simulink model "memristors_LSTM"  (R2020b)
settings: Solver=VariableStepAuto  StartTime=0.0  StopTime=3  RelTol=1e-3
libraries: simulink x17
(part 1 of 5)
settings Model: Creator=Иван  LastModifiedBy=Иван

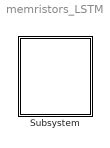
== system memristors_LSTM ==
  Subsystem : Subsystem

== system memristors_LSTM/Subsystem ==
  Add : Sum
  Display : Display
  Memristor crossbar1 : Subsystem
  Memristor crossbar2 : Subsystem
  Memristor crossbar4 : Subsystem
  Product : Product
  Product1 : Product
  Product2 : Product
  SIG : Subsystem
  SIG1 : Subsystem
  SIG2 : Subsystem
  TANH : Subsystem
  TANH1 : Subsystem
  s : Subsystem
  wires:
  Product/1 -> Add/1
  Product1/1 -> Add/2
  TANH1/1(Out1) -> Product2/2
  SIG2/1(Out1) -> Product2/1
  TANH/1(Out1) -> Product1/2
  SIG1/1(Out1) -> Product1/1
  Add/1 -> TANH1/1(In1)
  Memristor crossbar2/1(Out1) -> SIG1/1(In1)
  s/1(Out1) -> TANH/1(In1)
  Memristor crossbar4/1(Out1) -> SIG2/1(In1)
  Product2/1 -> Display/1
  SIG/1(Out1) -> Product/1
  Memristor crossbar1/1(Out1) -> SIG/1(In1)

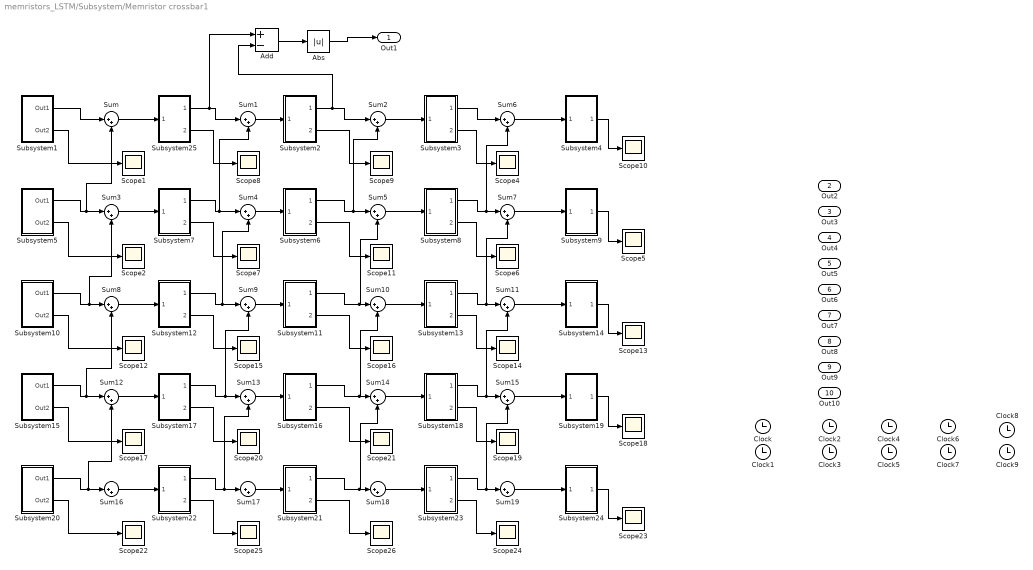
== system memristors_LSTM/Subsystem/Memristor crossbar1 ==
  Abs : Abs
  Add : Sum  Inputs=+-
  Clock{,1..9} (10 alike) : Clock
  Scope{1..2,4..26} (25 alike) : Scope
  Subsystem1 : Subsystem
  Subsystem10 : Subsystem
  Subsystem11 : Subsystem
  Subsystem12 : Subsystem
  Subsystem13 : Subsystem
  Subsystem14 : Subsystem
  Subsystem15 : Subsystem
  Subsystem16 : Subsystem
  Subsystem17 : Subsystem
  Subsystem18 : Subsystem
  Subsystem19 : Subsystem
  Subsystem2 : Subsystem
  Subsystem20 : Subsystem
  Subsystem21 : Subsystem
  Subsystem22 : Subsystem
  Subsystem23 : Subsystem
  Subsystem24 : Subsystem
  Subsystem25 : Subsystem
  Subsystem3 : Subsystem
  Subsystem4 : Subsystem
  Subsystem5 : Subsystem
  Subsystem6 : Subsystem
  Subsystem7 : Subsystem
  Subsystem8 : Subsystem
  Subsystem9 : Subsystem
  Sum{,1..19} (20 alike) : Sum  Inputs=|++
  Out1 : Outport
  Out2 : Outport  Port=2
  Out3 : Outport  Port=3
  Out4 : Outport  Port=4
  Out5 : Outport  Port=5
  Out6 : Outport  Port=6
  Out7 : Outport  Port=7
  Out8 : Outport  Port=8
  Out9 : Outport  Port=9
  Out10 : Outport  Port=10
  wires:
  Subsystem8/1(Out1) -> Sum6/2, Sum7/1
  Subsystem23/2(Out2) -> Scope24/1
  Subsystem6/1(Out1) -> Sum2/2, Sum5/1
  Subsystem20/1(Out1) -> Sum12/2, Sum16/1
  Subsystem1/1(Out1) -> Sum/1
  Subsystem2/1(Out1) -> Add/2, Sum2/1
  Subsystem17/2(Out2) -> Scope20/1
  Subsystem7/1(Out1) -> Sum1/2, Sum4/1
  Sum1/1 -> Subsystem2/1(In1)
  Subsystem18/1(Out1) -> Sum11/2, Sum15/1
  Subsystem6/2(Out2) -> Scope11/1
  Sum4/1 -> Subsystem6/1(In1)
  Subsystem5/2(Out2) -> Scope2/1
  Subsystem18/2(Out2) -> Scope19/1
  Subsystem11/1(Out1) -> Sum5/2, Sum10/1
  Sum18/1 -> Subsystem23/1(In1)
  Subsystem17/1(Out1) -> Sum9/2, Sum13/1
  Subsystem25/2(Out2) -> Scope8/1
  Subsystem13/2(Out2) -> Scope14/1
  Sum11/1 -> Subsystem14/1(In1)
  Subsystem21/2(Out2) -> Scope26/1
  Sum17/1 -> Subsystem21/1(In1)
  Sum/1 -> Subsystem25/1(In1)
  Subsystem2/2(Out2) -> Scope9/1
  Subsystem1/2(Out2) -> Scope1/1
  Subsystem20/2(Out2) -> Scope22/1
  Subsystem25/1(Out1) -> Add/1, Sum1/1
  Sum15/1 -> Subsystem19/1(In1)
  Sum8/1 -> Subsystem12/1(In1)
  Subsystem4/1(Out2) -> Scope10/1
  Subsystem5/1(Out1) -> Sum/2, Sum3/1
  Subsystem22/1(Out1) -> Sum13/2, Sum17/1
  Subsystem11/2(Out2) -> Scope16/1
  Sum5/1 -> Subsystem8/1(In1)
  Subsystem10/1(Out1) -> Sum3/2, Sum8/1
  Subsystem8/2(Out2) -> Scope6/1
  Subsystem7/2(Out2) -> Scope7/1
  Sum13/1 -> Subsystem16/1(In1)
  Subsystem10/2(Out2) -> Scope12/1
  Subsystem15/1(Out1) -> Sum8/2, Sum12/1
  Subsystem12/1(Out1) -> Sum4/2, Sum9/1
  Sum9/1 -> Subsystem11/1(In1)
  Sum6/1 -> Subsystem4/1(In1)
  Subsystem16/2(Out2) -> Scope21/1
  Subsystem13/1(Out1) -> Sum7/2, Sum11/1
  Sum19/1 -> Subsystem24/1(In1)
  Subsystem3/2(Out2) -> Scope4/1
  Sum7/1 -> Subsystem9/1(In1)
  Subsystem14/1(Out2) -> Scope13/1
  Subsystem16/1(Out1) -> Sum10/2, Sum14/1
  Subsystem3/1(Out1) -> Sum6/1
  Subsystem22/2(Out2) -> Scope25/1
  Sum12/1 -> Subsystem17/1(In1)
  Subsystem24/1(Out2) -> Scope23/1
  Subsystem9/1(Out2) -> Scope5/1
  Subsystem15/2(Out2) -> Scope17/1
  Sum10/1 -> Subsystem13/1(In1)
  Subsystem23/1(Out1) -> Sum15/2, Sum19/1
  Sum2/1 -> Subsystem3/1(In1)
  Subsystem12/2(Out2) -> Scope15/1
  Subsystem19/1(Out2) -> Scope18/1
  Sum14/1 -> Subsystem18/1(In1)
  Sum3/1 -> Subsystem7/1(In1)
  Subsystem21/1(Out1) -> Sum14/2, Sum18/1
  Sum16/1 -> Subsystem22/1(In1)
  Add/1 -> Abs/1
  Abs/1 -> Out1/1

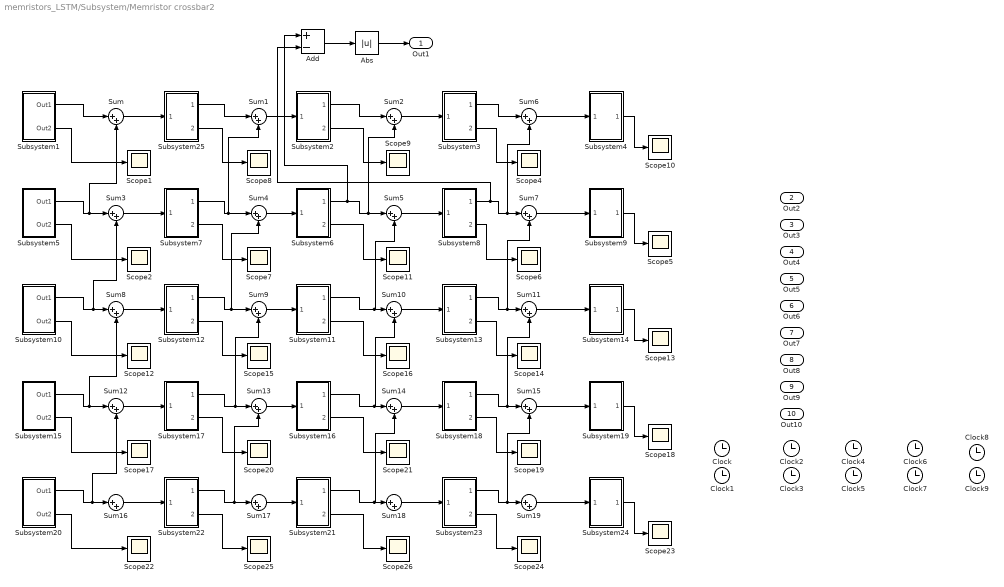
== system memristors_LSTM/Subsystem/Memristor crossbar2 ==
  Abs : Abs
  Add : Sum  Inputs=+-
  Clock{,1..9} (10 alike) : Clock
  Scope{1..2,4..26} (25 alike) : Scope
  Subsystem1 : Subsystem
  Subsystem10 : Subsystem
  Subsystem11 : Subsystem
  Subsystem12 : Subsystem
  Subsystem13 : Subsystem
  Subsystem14 : Subsystem
  Subsystem15 : Subsystem
  Subsystem16 : Subsystem
  Subsystem17 : Subsystem
  Subsystem18 : Subsystem
  Subsystem19 : Subsystem
  Subsystem2 : Subsystem
  Subsystem20 : Subsystem
  Subsystem21 : Subsystem
  Subsystem22 : Subsystem
  Subsystem23 : Subsystem
  Subsystem24 : Subsystem
  Subsystem25 : Subsystem
  Subsystem3 : Subsystem
  Subsystem4 : Subsystem
  Subsystem5 : Subsystem
  Subsystem6 : Subsystem
  Subsystem7 : Subsystem
  Subsystem8 : Subsystem
  Subsystem9 : Subsystem
  Sum{,1..19} (20 alike) : Sum  Inputs=|++
  Out1 : Outport
  Out2 : Outport  Port=2
  Out3 : Outport  Port=3
  Out4 : Outport  Port=4
  Out5 : Outport  Port=5
  Out6 : Outport  Port=6
  Out7 : Outport  Port=7
  Out8 : Outport  Port=8
  Out9 : Outport  Port=9
  Out10 : Outport  Port=10
  wires:
  Subsystem8/1(Out1) -> Add/2, Sum6/2, Sum7/1
  Subsystem23/2(Out2) -> Scope24/1
  Subsystem6/1(Out1) -> Add/1, Sum2/2, Sum5/1
  Subsystem20/1(Out1) -> Sum12/2, Sum16/1
  Subsystem1/1(Out1) -> Sum/1
  Subsystem2/1(Out1) -> Sum2/1
  Subsystem17/2(Out2) -> Scope20/1
  Subsystem7/1(Out1) -> Sum1/2, Sum4/1
  Sum1/1 -> Subsystem2/1(In1)
  Subsystem18/1(Out1) -> Sum11/2, Sum15/1
  Subsystem6/2(Out2) -> Scope11/1
  Sum4/1 -> Subsystem6/1(In1)
  Subsystem5/2(Out2) -> Scope2/1
  Subsystem18/2(Out2) -> Scope19/1
  Subsystem11/1(Out1) -> Sum5/2, Sum10/1
  Sum18/1 -> Subsystem23/1(In1)
  Subsystem17/1(Out1) -> Sum9/2, Sum13/1
  Subsystem25/2(Out2) -> Scope8/1
  Subsystem13/2(Out2) -> Scope14/1
  Sum11/1 -> Subsystem14/1(In1)
  Subsystem21/2(Out2) -> Scope26/1
  Sum17/1 -> Subsystem21/1(In1)
  Sum/1 -> Subsystem25/1(In1)
  Subsystem2/2(Out2) -> Scope9/1
  Subsystem1/2(Out2) -> Scope1/1
  Subsystem20/2(Out2) -> Scope22/1
  Subsystem25/1(Out1) -> Sum1/1
  Sum15/1 -> Subsystem19/1(In1)
  Sum8/1 -> Subsystem12/1(In1)
  Subsystem4/1(Out2) -> Scope10/1
  Subsystem5/1(Out1) -> Sum/2, Sum3/1
  Subsystem22/1(Out1) -> Sum13/2, Sum17/1
  Subsystem11/2(Out2) -> Scope16/1
  Sum5/1 -> Subsystem8/1(In1)
  Subsystem10/1(Out1) -> Sum3/2, Sum8/1
  Subsystem8/2(Out2) -> Scope6/1
  Subsystem7/2(Out2) -> Scope7/1
  Sum13/1 -> Subsystem16/1(In1)
  Subsystem10/2(Out2) -> Scope12/1
  Subsystem15/1(Out1) -> Sum8/2, Sum12/1
  Subsystem12/1(Out1) -> Sum4/2, Sum9/1
  Sum9/1 -> Subsystem11/1(In1)
  Sum6/1 -> Subsystem4/1(In1)
  Subsystem16/2(Out2) -> Scope21/1
  Subsystem13/1(Out1) -> Sum7/2, Sum11/1
  Sum19/1 -> Subsystem24/1(In1)
  Subsystem3/2(Out2) -> Scope4/1
  Sum7/1 -> Subsystem9/1(In1)
  Subsystem14/1(Out2) -> Scope13/1
  Subsystem16/1(Out1) -> Sum10/2, Sum14/1
  Subsystem3/1(Out1) -> Sum6/1
  Subsystem22/2(Out2) -> Scope25/1
  Sum12/1 -> Subsystem17/1(In1)
  Subsystem24/1(Out2) -> Scope23/1
  Subsystem9/1(Out2) -> Scope5/1
  Subsystem15/2(Out2) -> Scope17/1
  Sum10/1 -> Subsystem13/1(In1)
  Subsystem23/1(Out1) -> Sum15/2, Sum19/1
  Sum2/1 -> Subsystem3/1(In1)
  Subsystem12/2(Out2) -> Scope15/1
  Subsystem19/1(Out2) -> Scope18/1
  Sum14/1 -> Subsystem18/1(In1)
  Sum3/1 -> Subsystem7/1(In1)
  Subsystem21/1(Out1) -> Sum14/2, Sum18/1
  Sum16/1 -> Subsystem22/1(In1)
  Add/1 -> Abs/1
  Abs/1 -> Out1/1

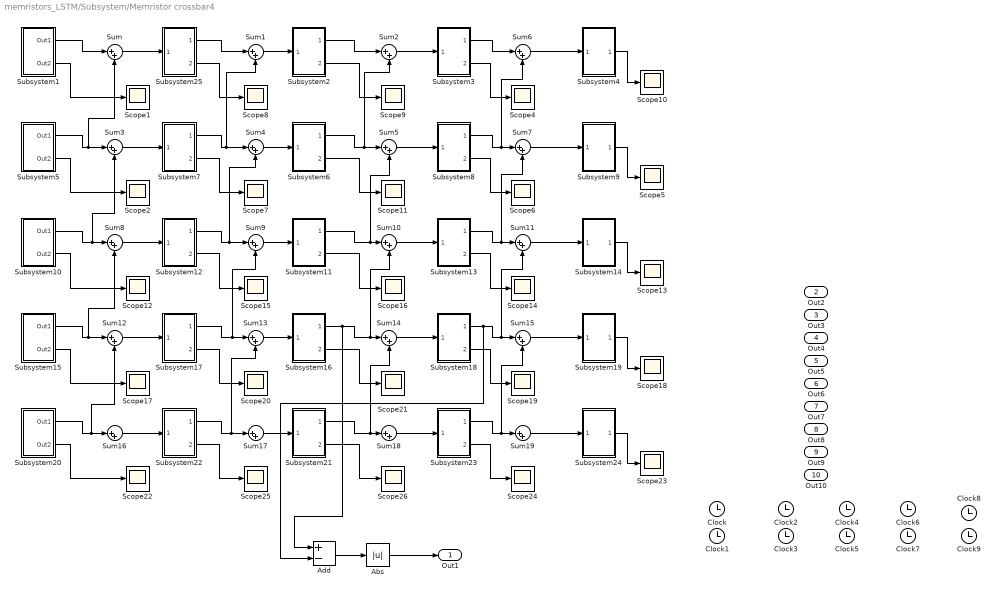
== system memristors_LSTM/Subsystem/Memristor crossbar4 ==
  Abs : Abs
  Add : Sum  Inputs=+-
  Clock{,1..9} (10 alike) : Clock
  Scope{1..2,4..26} (25 alike) : Scope
  Subsystem1 : Subsystem
  Subsystem10 : Subsystem
  Subsystem11 : Subsystem
  Subsystem12 : Subsystem
  Subsystem13 : Subsystem
  Subsystem14 : Subsystem
  Subsystem15 : Subsystem
  Subsystem16 : Subsystem
  Subsystem17 : Subsystem
  Subsystem18 : Subsystem
  Subsystem19 : Subsystem
  Subsystem2 : Subsystem
  Subsystem20 : Subsystem
  Subsystem21 : Subsystem
  Subsystem22 : Subsystem
  Subsystem23 : Subsystem
  Subsystem24 : Subsystem
  Subsystem25 : Subsystem
  Subsystem3 : Subsystem
  Subsystem4 : Subsystem
  Subsystem5 : Subsystem
  Subsystem6 : Subsystem
  Subsystem7 : Subsystem
  Subsystem8 : Subsystem
  Subsystem9 : Subsystem
  Sum{,1..19} (20 alike) : Sum  Inputs=|++
  Out1 : Outport
  Out2 : Outport  Port=2
  Out3 : Outport  Port=3
  Out4 : Outport  Port=4
  Out5 : Outport  Port=5
  Out6 : Outport  Port=6
  Out7 : Outport  Port=7
  Out8 : Outport  Port=8
  Out9 : Outport  Port=9
  Out10 : Outport  Port=10
  wires:
  Subsystem8/1(Out1) -> Sum6/2, Sum7/1
  Subsystem23/2(Out2) -> Scope24/1
  Subsystem6/1(Out1) -> Sum2/2, Sum5/1
  Subsystem20/1(Out1) -> Sum12/2, Sum16/1
  Subsystem1/1(Out1) -> Sum/1
  Subsystem2/1(Out1) -> Sum2/1
  Subsystem17/2(Out2) -> Scope20/1
  Subsystem7/1(Out1) -> Sum1/2, Sum4/1
  Sum1/1 -> Subsystem2/1(In1)
  Subsystem18/1(Out1) -> Add/2, Sum11/2, Sum15/1
  Subsystem6/2(Out2) -> Scope11/1
  Sum4/1 -> Subsystem6/1(In1)
  Subsystem5/2(Out2) -> Scope2/1
  Subsystem18/2(Out2) -> Scope19/1
  Subsystem11/1(Out1) -> Sum5/2, Sum10/1
  Sum18/1 -> Subsystem23/1(In1)
  Subsystem17/1(Out1) -> Sum9/2, Sum13/1
  Subsystem25/2(Out2) -> Scope8/1
  Subsystem13/2(Out2) -> Scope14/1
  Sum11/1 -> Subsystem14/1(In1)
  Subsystem21/2(Out2) -> Scope26/1
  Sum17/1 -> Subsystem21/1(In1)
  Sum/1 -> Subsystem25/1(In1)
  Subsystem2/2(Out2) -> Scope9/1
  Subsystem1/2(Out2) -> Scope1/1
  Subsystem20/2(Out2) -> Scope22/1
  Subsystem25/1(Out1) -> Sum1/1
  Sum15/1 -> Subsystem19/1(In1)
  Sum8/1 -> Subsystem12/1(In1)
  Subsystem4/1(Out2) -> Scope10/1
  Subsystem5/1(Out1) -> Sum/2, Sum3/1
  Subsystem22/1(Out1) -> Sum13/2, Sum17/1
  Subsystem11/2(Out2) -> Scope16/1
  Sum5/1 -> Subsystem8/1(In1)
  Subsystem10/1(Out1) -> Sum3/2, Sum8/1
  Subsystem8/2(Out2) -> Scope6/1
  Subsystem7/2(Out2) -> Scope7/1
  Sum13/1 -> Subsystem16/1(In1)
  Subsystem10/2(Out2) -> Scope12/1
  Subsystem15/1(Out1) -> Sum8/2, Sum12/1
  Subsystem12/1(Out1) -> Sum4/2, Sum9/1
  Sum9/1 -> Subsystem11/1(In1)
  Sum6/1 -> Subsystem4/1(In1)
  Subsystem16/2(Out2) -> Scope21/1
  Subsystem13/1(Out1) -> Sum7/2, Sum11/1
  Sum19/1 -> Subsystem24/1(In1)
  Subsystem3/2(Out2) -> Scope4/1
  Sum7/1 -> Subsystem9/1(In1)
  Subsystem14/1(Out2) -> Scope13/1
  Subsystem16/1(Out1) -> Add/1, Sum10/2, Sum14/1
  Subsystem3/1(Out1) -> Sum6/1
  Subsystem22/2(Out2) -> Scope25/1
  Sum12/1 -> Subsystem17/1(In1)
  Subsystem24/1(Out2) -> Scope23/1
  Subsystem9/1(Out2) -> Scope5/1
  Subsystem15/2(Out2) -> Scope17/1
  Sum10/1 -> Subsystem13/1(In1)
  Subsystem23/1(Out1) -> Sum15/2, Sum19/1
  Sum2/1 -> Subsystem3/1(In1)
  Subsystem12/2(Out2) -> Scope15/1
  Subsystem19/1(Out2) -> Scope18/1
  Sum14/1 -> Subsystem18/1(In1)
  Sum3/1 -> Subsystem7/1(In1)
  Subsystem21/1(Out1) -> Sum14/2, Sum18/1
  Sum16/1 -> Subsystem22/1(In1)
  Add/1 -> Abs/1
  Abs/1 -> Out1/1

== system memristors_LSTM/Subsystem/SIG ==
  In1 : Inport
  Add4 : Sum
  Constant1 : Constant
  Constant2 : Constant
  Divide2 : Product  Inputs=*/
  Integrator2 : Integrator  InitialCondition=-10
  Math Function2 : Math  Operator=reciprocal  SaturateOnIntegerOverflow=on
  Math Function3 : Math  SaturateOnIntegerOverflow=on
  Product : Product
  Ramp : simulink/Sources/Ramp  slope=1  start=-4  InitialOutput=0
  Scope1 : Scope
  Out1 : Outport
  wires:
  Constant2/1 -> Add4/1
  Divide2/1 -> Product/1
  Math Function2/1 -> Add4/2
  Math Function3/1 -> Math Function2/1
  Add4/1 -> Divide2/2
  Constant1/1 -> Divide2/1
  Integrator2/1 -> Math Function3/1
  Ramp/1 -> Scope1/1, Integrator2/1
  In1/1 -> Product/2
  Product/1 -> Out1/1

== system memristors_LSTM/Subsystem/SIG1 ==
  In1 : Inport
  Add4 : Sum
  Constant1 : Constant
  Constant2 : Constant
  Divide2 : Product  Inputs=*/
  Integrator2 : Integrator  InitialCondition=-10
  Math Function2 : Math  Operator=reciprocal  SaturateOnIntegerOverflow=on
  Math Function3 : Math  SaturateOnIntegerOverflow=on
  Product : Product
  Ramp : simulink/Sources/Ramp  slope=1  start=-4  InitialOutput=0
  Out1 : Outport
  wires:
  Constant2/1 -> Add4/1
  Math Function2/1 -> Add4/2
  Math Function3/1 -> Math Function2/1
  Integrator2/1 -> Math Function3/1
  Add4/1 -> Divide2/2
  Constant1/1 -> Divide2/1
  Ramp/1 -> Integrator2/1
  Divide2/1 -> Product/2
  In1/1 -> Product/1  "In"
  Product/1 -> Out1/1

== system memristors_LSTM/Subsystem/SIG2 ==
  In1 : Inport
  Add4 : Sum
  Constant1 : Constant
  Constant2 : Constant
  Divide2 : Product  Inputs=*/
  Integrator2 : Integrator  InitialCondition=-10
  Math Function2 : Math  Operator=reciprocal  SaturateOnIntegerOverflow=on
  Math Function3 : Math  SaturateOnIntegerOverflow=on
  Product : Product
  Ramp : simulink/Sources/Ramp  slope=1  start=-4  InitialOutput=0
  Out1 : Outport
  wires:
  Constant2/1 -> Add4/1
  Math Function2/1 -> Add4/2
  Math Function3/1 -> Math Function2/1
  Integrator2/1 -> Math Function3/1
  Add4/1 -> Divide2/2
  Constant1/1 -> Divide2/1
  Ramp/1 -> Integrator2/1
  Divide2/1 -> Product/2
  Product/1 -> Out1/1
  In1/1 -> Product/1

== system memristors_LSTM/Subsystem/TANH ==
  In1 : Inport
  Atanh1 : Trigonometry  Operator=tanh
  Integrator1 : Integrator  InitialCondition=-4
  Product : Product
  Ramp : simulink/Sources/Ramp  slope=1  start=-4  InitialOutput=0
  Out1 : Outport
  wires:
  Ramp/1 -> Integrator1/1
  Integrator1/1 -> Atanh1/1
  Product/1 -> Out1/1
  Atanh1/1 -> Product/2
  In1/1 -> Product/1

== system memristors_LSTM/Subsystem/TANH1 ==
  In1 : Inport
  Atanh1 : Trigonometry  Operator=tanh
  Integrator1 : Integrator  InitialCondition=-4
  Product1 : Product
  Ramp : simulink/Sources/Ramp  slope=1  start=-4  InitialOutput=0
  Scope : Scope
  Out1 : Outport
  wires:
  Atanh1/1 -> Scope/1, Product1/2
  Integrator1/1 -> Atanh1/1
  Ramp/1 -> Integrator1/1
  Product1/1 -> Out1/1
  In1/1 -> Product1/1

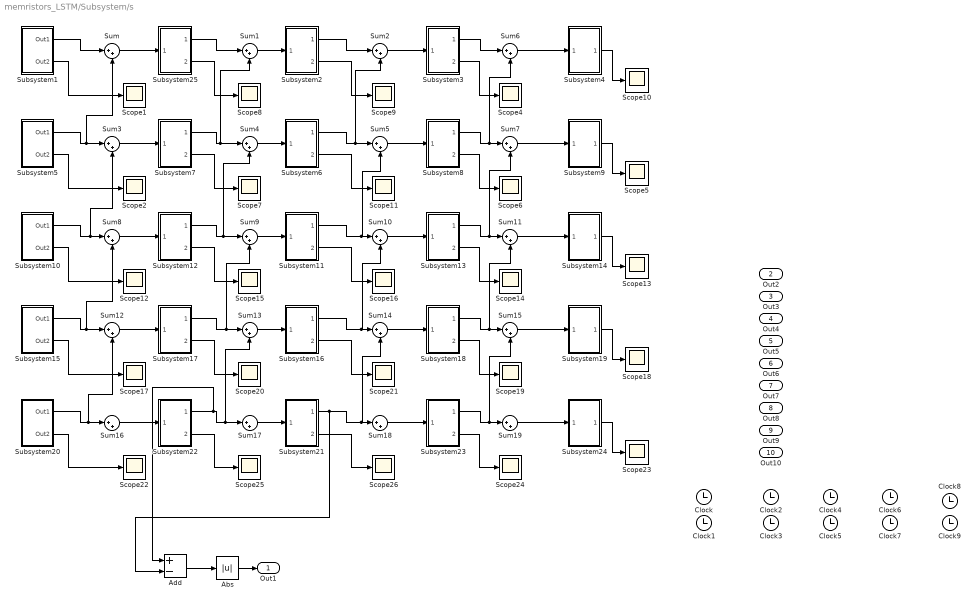
== system memristors_LSTM/Subsystem/s ==
  Abs : Abs
  Add : Sum  Inputs=+-
  Clock{,1..9} (10 alike) : Clock
  Scope{1..2,4..26} (25 alike) : Scope
  Subsystem1 : Subsystem
  Subsystem10 : Subsystem
  Subsystem11 : Subsystem
  Subsystem12 : Subsystem
  Subsystem13 : Subsystem
  Subsystem14 : Subsystem
  Subsystem15 : Subsystem
  Subsystem16 : Subsystem
  Subsystem17 : Subsystem
  Subsystem18 : Subsystem
  Subsystem19 : Subsystem
  Subsystem2 : Subsystem
  Subsystem20 : Subsystem
  Subsystem21 : Subsystem
  Subsystem22 : Subsystem
  Subsystem23 : Subsystem
  Subsystem24 : Subsystem
  Subsystem25 : Subsystem
  Subsystem3 : Subsystem
  Subsystem4 : Subsystem
  Subsystem5 : Subsystem
  Subsystem6 : Subsystem
  Subsystem7 : Subsystem
  Subsystem8 : Subsystem
  Subsystem9 : Subsystem
  Sum{,1..19} (20 alike) : Sum  Inputs=|++
  Out1 : Outport
  Out2 : Outport  Port=2
  Out3 : Outport  Port=3
  Out4 : Outport  Port=4
  Out5 : Outport  Port=5
  Out6 : Outport  Port=6
  Out7 : Outport  Port=7
  Out8 : Outport  Port=8
  Out9 : Outport  Port=9
  Out10 : Outport  Port=10
  wires:
  Subsystem8/1(Out1) -> Sum6/2, Sum7/1
  Subsystem23/2(Out2) -> Scope24/1
  Subsystem6/1(Out1) -> Sum2/2, Sum5/1
  Subsystem20/1(Out1) -> Sum12/2, Sum16/1
  Subsystem1/1(Out1) -> Sum/1
  Subsystem2/1(Out1) -> Sum2/1
  Subsystem17/2(Out2) -> Scope20/1
  Subsystem7/1(Out1) -> Sum1/2, Sum4/1
  Sum1/1 -> Subsystem2/1(In1)
  Subsystem18/1(Out1) -> Sum11/2, Sum15/1
  Subsystem6/2(Out2) -> Scope11/1
  Sum4/1 -> Subsystem6/1(In1)
  Subsystem5/2(Out2) -> Scope2/1
  Subsystem18/2(Out2) -> Scope19/1
  Subsystem11/1(Out1) -> Sum5/2, Sum10/1
  Sum18/1 -> Subsystem23/1(In1)
  Subsystem17/1(Out1) -> Sum9/2, Sum13/1
  Subsystem25/2(Out2) -> Scope8/1
  Subsystem13/2(Out2) -> Scope14/1
  Sum11/1 -> Subsystem14/1(In1)
  Subsystem21/2(Out2) -> Scope26/1
  Sum17/1 -> Subsystem21/1(In1)
  Sum/1 -> Subsystem25/1(In1)
  Subsystem2/2(Out2) -> Scope9/1
  Subsystem1/2(Out2) -> Scope1/1
  Subsystem20/2(Out2) -> Scope22/1
  Subsystem25/1(Out1) -> Sum1/1
  Sum15/1 -> Subsystem19/1(In1)
  Sum8/1 -> Subsystem12/1(In1)
  Subsystem4/1(Out2) -> Scope10/1
  Subsystem5/1(Out1) -> Sum/2, Sum3/1
  Subsystem22/1(Out1) -> Add/1, Sum13/2, Sum17/1
  Subsystem11/2(Out2) -> Scope16/1
  Sum5/1 -> Subsystem8/1(In1)
  Subsystem10/1(Out1) -> Sum3/2, Sum8/1
  Subsystem8/2(Out2) -> Scope6/1
  Subsystem7/2(Out2) -> Scope7/1
  Sum13/1 -> Subsystem16/1(In1)
  Subsystem10/2(Out2) -> Scope12/1
  Subsystem15/1(Out1) -> Sum8/2, Sum12/1
  Subsystem12/1(Out1) -> Sum4/2, Sum9/1
  Sum9/1 -> Subsystem11/1(In1)
  Sum6/1 -> Subsystem4/1(In1)
  Subsystem16/2(Out2) -> Scope21/1
  Subsystem13/1(Out1) -> Sum7/2, Sum11/1
  Sum19/1 -> Subsystem24/1(In1)
  Subsystem3/2(Out2) -> Scope4/1
  Sum7/1 -> Subsystem9/1(In1)
  Subsystem14/1(Out2) -> Scope13/1
  Subsystem16/1(Out1) -> Sum10/2, Sum14/1
  Subsystem3/1(Out1) -> Sum6/1
  Subsystem22/2(Out2) -> Scope25/1
  Sum12/1 -> Subsystem17/1(In1)
  Subsystem24/1(Out2) -> Scope23/1
  Subsystem9/1(Out2) -> Scope5/1
  Subsystem15/2(Out2) -> Scope17/1
  Sum10/1 -> Subsystem13/1(In1)
  Subsystem23/1(Out1) -> Sum15/2, Sum19/1
  Sum2/1 -> Subsystem3/1(In1)
  Subsystem12/2(Out2) -> Scope15/1
  Subsystem19/1(Out2) -> Scope18/1
  Sum14/1 -> Subsystem18/1(In1)
  Sum3/1 -> Subsystem7/1(In1)
  Subsystem21/1(Out1) -> Add/2, Sum14/2, Sum18/1
  Sum16/1 -> Subsystem22/1(In1)
  Add/1 -> Abs/1
  Abs/1 -> Out1/1

== system memristors_LSTM/Subsystem/Memristor crossbar1/Subsystem1 ==
  note: Memristor
  note: k
  note: for I-V
  note: Rmem
  note: f(x)
  note: for x
  note: for processing
  " V" : Sin  Amplitude=0.1  Frequency=0.5  SampleTime=0
  2p : Gain  Gain=2
  2x : Gain  Gain=2
  Add : Sum  Inputs=-+
  Add1 : Sum
  Add2 : Sum  Inputs=-+
  Add3 : Sum  Inputs=+-
  Constant : Constant
  Constant10 : Constant  Value=0
  Constant4 : Constant
  Constant9 : Constant
  D : Constant  Value=10^(-8)
  Divide : Product  Inputs=*/
  Divide1 : Product  Inputs=**/
  Gain2 : Gain
  I-t : Scope
  Integrator : Integrator
  Integrator Initial condition source : Integrator  InitialConditionSource=external
  Math Function : Math  Operator=pow  SaturateOnIntegerOverflow=on
  Math Function1 : Math  Operator=square  SaturateOnIntegerOverflow=on
  Product1 : Product
  Product2 : Product
  Product3 : Product  Inputs=3
  Product4 : Product
  R_off : Constant  Value=20000
  R_on : Constant  Value=100
  R_on1 : Constant  Value=100
  Switch : Switch  Threshold=1
  Switch1 : Switch
  V-t : Scope
  XY Graph : simulink/Sinks/XY Graph  xmin=-0.05  xmax=0.05  ymin=-0.01  ymax=0.01  st=-1
  p : Constant  Value=10
  x-t : Scope
  x0 : Constant  Value=0.7
  𝜇_𝑣 : Constant  Value=10^(-14)
  Out1 : Outport
  Out2 : Outport  Port=2
  wires:
  Constant9/1 -> Switch/1
  Switch/1 -> Switch1/2, Switch1/1
  R_on/1 -> Divide1/1
  Integrator Initial condition source/1 -> Switch/3, Switch/2, x-t/1
  Integrator/1 -> Divide/1, Product4/2
  2p/1 -> Math Function/2
  Divide/1 -> XY Graph/2, I-t/1, Product3/1
  Switch1/1 -> Product2/2, Add/1, 2x/1
  𝜇_𝑣/1 -> Divide1/2
  Gain2/1 -> Integrator/1
  Math Function/1 -> Add3/2
  Add/1 -> Product1/1
  R_on1/1 -> Product2/1
  Constant/1 -> Add/2
  p/1 -> 2p/1
  D/1 -> Math Function1/1
  Divide1/1 -> Product3/3
  2x/1 -> Add2/2
  Product1/1 -> Add1/2
  R_off/1 -> Product1/2
  Add2/1 -> Math Function/1
  Constant4/1 -> Add3/1, Add2/1
  Product4/1 -> Out1/1, XY Graph/1, Out2/1, V-t/1
  Product2/1 -> Add1/1
  x0/1 -> Integrator Initial condition source/2
  Constant10/1 -> Switch1/3
  Product3/1 -> Integrator Initial condition source/1
  Add1/1 -> Divide/2
  Add3/1 -> Product3/2
  Math Function1/1 -> Divide1/3
  " V"/1 -> Gain2/1, Product4/1

== system memristors_LSTM/Subsystem/Memristor crossbar1/Subsystem10 ==
  note: Memristor
  note: k
  note: for I-V
  note: Rmem
  note: f(x)
  note: for x
  note: for processing
  " V" : Sin  Amplitude=0.1  Frequency=0.5  SampleTime=0
  2p : Gain  Gain=2
  2x : Gain  Gain=2
  Add : Sum  Inputs=-+
  Add1 : Sum
  Add2 : Sum  Inputs=-+
  Add3 : Sum  Inputs=+-
  Constant : Constant
  Constant10 : Constant  Value=0
  Constant4 : Constant
  Constant9 : Constant
  D : Constant  Value=10^(-8)
  Divide : Product  Inputs=*/
  Divide1 : Product  Inputs=**/
  Gain2 : Gain  Gain=0.5
  I-t : Scope
  Integrator : Integrator
  Integrator Initial condition source : Integrator  InitialConditionSource=external
  Math Function : Math  Operator=pow  SaturateOnIntegerOverflow=on
  Math Function1 : Math  Operator=square  SaturateOnIntegerOverflow=on
  Product1 : Product
  Product2 : Product
  Product3 : Product  Inputs=3
  Product4 : Product
  R_off : Constant  Value=20000
  R_on : Constant  Value=100
  R_on1 : Constant  Value=100
  Switch : Switch  Threshold=1
  Switch1 : Switch
  V-t : Scope
  p : Constant  Value=10
  x-t : Scope
  x0 : Constant  Value=0.7
  𝜇_𝑣 : Constant  Value=10^(-14)
  Out1 : Outport
  Out2 : Outport  Port=2
  wires:
  Constant9/1 -> Switch/1
  Switch/1 -> Switch1/2, Switch1/1
  R_on/1 -> Divide1/1
  Integrator Initial condition source/1 -> Switch/3, Switch/2, x-t/1
  Integrator/1 -> Divide/1, Product4/2
  2p/1 -> Math Function/2
  Divide/1 -> I-t/1, Product3/1
  Switch1/1 -> Product2/2, Add/1, 2x/1
  𝜇_𝑣/1 -> Divide1/2
  Gain2/1 -> Integrator/1
  Math Function/1 -> Add3/2
  Add/1 -> Product1/1
  R_on1/1 -> Product2/1
  Constant/1 -> Add/2
  p/1 -> 2p/1
  D/1 -> Math Function1/1
  Divide1/1 -> Product3/3
  2x/1 -> Add2/2
  Product1/1 -> Add1/2
  R_off/1 -> Product1/2
  Add2/1 -> Math Function/1
  Constant4/1 -> Add3/1, Add2/1
  Product4/1 -> Out1/1, Out2/1, V-t/1
  Product2/1 -> Add1/1
  x0/1 -> Integrator Initial condition source/2
  Constant10/1 -> Switch1/3
  Product3/1 -> Integrator Initial condition source/1
  Add1/1 -> Divide/2
  Add3/1 -> Product3/2
  Math Function1/1 -> Divide1/3
  " V"/1 -> Gain2/1, Product4/1

== system memristors_LSTM/Subsystem/Memristor crossbar1/Subsystem11 ==
  note: Memristor
  note: k
  note: for I-V
  note: Rmem
  note: f(x)
  note: for x
  note: for processing
  In1 : Inport
  " V" : Sin  Frequency=0.5  SampleTime=0
  2p : Gain  Gain=2
  2x : Gain  Gain=2
  Add : Sum  Inputs=-+
  Add1 : Sum
  Add2 : Sum  Inputs=-+
  Add3 : Sum  Inputs=+-
  Add4 : Sum
  Constant : Constant
  Constant10 : Constant  Value=0
  Constant4 : Constant
  Constant9 : Constant
  D : Constant  Value=10^(-8)
  Divide : Product  Inputs=*/
  Divide1 : Product  Inputs=**/
  Gain2 : Gain  Gain=0.5
  I-t : Scope
  Integrator : Integrator
  Integrator Initial condition source : Integrator  InitialConditionSource=external
  Math Function : Math  Operator=pow  SaturateOnIntegerOverflow=on
  Math Function1 : Math  Operator=square  SaturateOnIntegerOverflow=on
  Product1 : Product
  Product2 : Product
  Product3 : Product  Inputs=3
  Product4 : Product
  R_off : Constant  Value=20000
  R_on : Constant  Value=100
  R_on1 : Constant  Value=100
  Switch : Switch  Threshold=1
  Switch1 : Switch
  V-t : Scope
  p : Constant  Value=10
  x-t : Scope
  x0 : Constant  Value=0.7
  𝜇_𝑣 : Constant  Value=10^(-14)
  Out1 : Outport
  Out2 : Outport  Port=2
  wires:
  Constant9/1 -> Switch/1
  Switch/1 -> Switch1/2, Switch1/1
  R_on/1 -> Divide1/1
  Integrator Initial condition source/1 -> Switch/3, Switch/2, x-t/1
  2p/1 -> Math Function/2
  Divide/1 -> I-t/1, Product3/1
  Switch1/1 -> Product2/2, Add/1, 2x/1
  𝜇_𝑣/1 -> Divide1/2
  Gain2/1 -> Integrator/1
  Math Function/1 -> Add3/2
  Add/1 -> Product1/1
  R_on1/1 -> Product2/1
  Constant/1 -> Add/2
  p/1 -> 2p/1
  D/1 -> Math Function1/1
  Divide1/1 -> Product3/3
  2x/1 -> Add2/2
  Product1/1 -> Add1/2
  R_off/1 -> Product1/2
  Add2/1 -> Math Function/1
  Constant4/1 -> Add3/1, Add2/1
  Product4/1 -> Out1/1, Out2/1, V-t/1
  Product2/1 -> Add1/1
  x0/1 -> Integrator Initial condition source/2
  Constant10/1 -> Switch1/3
  Product3/1 -> Integrator Initial condition source/1
  Add1/1 -> Divide/2
  Add3/1 -> Product3/2
  Math Function1/1 -> Divide1/3
  " V"/1 -> Add4/2
  In1/1 -> Add4/1
  Add4/1 -> Product4/1, Gain2/1
  Integrator/1 -> Divide/1, Product4/2

== system memristors_LSTM/Subsystem/Memristor crossbar1/Subsystem12 ==
  note: k
  note: for I-V
  note: Rmem
  note: f(x)
  note: for x
  note: for processing
  In1 : Inport
  " V" : Sin  Frequency=0.5  SampleTime=0
  2p : Gain  Gain=2
  2x : Gain  Gain=2
  Add : Sum  Inputs=-+
  Add1 : Sum
  Add2 : Sum  Inputs=-+
  Add3 : Sum  Inputs=+-
  Add4 : Sum
  Constant : Constant
  Constant10 : Constant  Value=0
  Constant4 : Constant
  Constant9 : Constant
  D : Constant  Value=10^(-8)
  Divide : Product  Inputs=*/
  Divide1 : Product  Inputs=**/
  Gain2 : Gain  Gain=0.5
  I-t : Scope
  Integrator : Integrator
  Integrator Initial condition source : Integrator  InitialConditionSource=external
  Math Function : Math  Operator=pow  SaturateOnIntegerOverflow=on
  Math Function1 : Math  Operator=square  SaturateOnIntegerOverflow=on
  Product1 : Product
  Product2 : Product
  Product3 : Product  Inputs=3
  Product4 : Product
  R_off : Constant  Value=20000
  R_on : Constant  Value=100
  R_on1 : Constant  Value=100
  Switch : Switch  Threshold=1
  Switch1 : Switch
  V-t : Scope
  p : Constant  Value=10
  x-t : Scope
  x0 : Constant  Value=0.7
  𝜇_𝑣 : Constant  Value=10^(-14)
  Out1 : Outport
  Out2 : Outport  Port=2
  wires:
  Constant9/1 -> Switch/1
  Switch/1 -> Switch1/2, Switch1/1
  R_on/1 -> Divide1/1
  Integrator Initial condition source/1 -> Switch/3, Switch/2, x-t/1
  Integrator/1 -> Divide/1, Product4/2
  2p/1 -> Math Function/2
  Divide/1 -> I-t/1, Product3/1
  Switch1/1 -> Product2/2, Add/1, 2x/1
  𝜇_𝑣/1 -> Divide1/2
  Gain2/1 -> Integrator/1
  Math Function/1 -> Add3/2
  Add/1 -> Product1/1
  R_on1/1 -> Product2/1
  Constant/1 -> Add/2
  p/1 -> 2p/1
  D/1 -> Math Function1/1
  Divide1/1 -> Product3/3
  2x/1 -> Add2/2
  Product1/1 -> Add1/2
  R_off/1 -> Product1/2
  Add2/1 -> Math Function/1
  Constant4/1 -> Add3/1, Add2/1
  Product2/1 -> Add1/1
  x0/1 -> Integrator Initial condition source/2
  Constant10/1 -> Switch1/3
  Product3/1 -> Integrator Initial condition source/1
  Add1/1 -> Divide/2
  Add3/1 -> Product3/2
  Math Function1/1 -> Divide1/3
  " V"/1 -> Add4/2
  In1/1 -> Add4/1
  Add4/1 -> Product4/1, Gain2/1
  Product4/1 -> Out1/1, Out2/1, V-t/1

== system memristors_LSTM/Subsystem/Memristor crossbar1/Subsystem13 ==
  note: Memristor
  note: k
  note: for I-V
  note: Rmem
  note: f(x)
  note: for x
  note: for processing
  In1 : Inport
  " V" : Sin  Frequency=0.5  SampleTime=0
  2p : Gain  Gain=2
  2x : Gain  Gain=2
  Add : Sum  Inputs=-+
  Add1 : Sum
  Add2 : Sum  Inputs=-+
  Add3 : Sum  Inputs=+-
  Add4 : Sum
  Constant : Constant
  Constant10 : Constant  Value=0
  Constant4 : Constant
  Constant9 : Constant
  D : Constant  Value=10^(-8)
  Divide : Product  Inputs=*/
  Divide1 : Product  Inputs=**/
  Gain2 : Gain  Gain=0.5
  I-t : Scope
  Integrator : Integrator
  Integrator Initial condition source : Integrator  InitialConditionSource=external
  Math Function : Math  Operator=pow  SaturateOnIntegerOverflow=on
  Math Function1 : Math  Operator=square  SaturateOnIntegerOverflow=on
  Product1 : Product
  Product2 : Product
  Product3 : Product  Inputs=3
  Product4 : Product
  R_off : Constant  Value=20000
  R_on : Constant  Value=100
  R_on1 : Constant  Value=100
  Switch : Switch  Threshold=1
  Switch1 : Switch
  V-t : Scope
  p : Constant  Value=10
  x-t : Scope
  x0 : Constant  Value=0.7
  𝜇_𝑣 : Constant  Value=10^(-14)
  Out1 : Outport
  Out2 : Outport  Port=2
  wires:
  Constant9/1 -> Switch/1
  Switch/1 -> Switch1/2, Switch1/1
  R_on/1 -> Divide1/1
  Integrator Initial condition source/1 -> Switch/3, Switch/2, x-t/1
  Integrator/1 -> Divide/1, Product4/2
  2p/1 -> Math Function/2
  Divide/1 -> I-t/1, Product3/1
  Switch1/1 -> Product2/2, Add/1, 2x/1
  𝜇_𝑣/1 -> Divide1/2
  Gain2/1 -> Integrator/1
  Math Function/1 -> Add3/2
  Add/1 -> Product1/1
  R_on1/1 -> Product2/1
  Constant/1 -> Add/2
  p/1 -> 2p/1
  D/1 -> Math Function1/1
  Divide1/1 -> Product3/3
  2x/1 -> Add2/2
  Product1/1 -> Add1/2
  R_off/1 -> Product1/2
  Add2/1 -> Math Function/1
  Constant4/1 -> Add3/1, Add2/1
  Product4/1 -> Out1/1, Out2/1, V-t/1
  Product2/1 -> Add1/1
  x0/1 -> Integrator Initial condition source/2
  Constant10/1 -> Switch1/3
  Product3/1 -> Integrator Initial condition source/1
  Add1/1 -> Divide/2
  Add3/1 -> Product3/2
  Math Function1/1 -> Divide1/3
  " V"/1 -> Add4/2
  In1/1 -> Add4/1
  Add4/1 -> Product4/1, Gain2/1

== system memristors_LSTM/Subsystem/Memristor crossbar1/Subsystem14 ==
  note: Memristor
  note: k
  note: for I-V
  note: Rmem
  note: f(x)
  note: for x
  note: for processing
  In1 : Inport
  " V" : Sin  Frequency=0.5  SampleTime=0
  2p : Gain  Gain=2
  2x : Gain  Gain=2
  Add : Sum  Inputs=-+
  Add1 : Sum
  Add2 : Sum  Inputs=-+
  Add3 : Sum  Inputs=+-
  Add4 : Sum
  Constant : Constant
  Constant10 : Constant  Value=0
  Constant4 : Constant
  Constant9 : Constant
  D : Constant  Value=10^(-8)
  Divide : Product  Inputs=*/
  Divide1 : Product  Inputs=**/
  Gain2 : Gain  Gain=0.5
  I-t : Scope
  Integrator : Integrator
  Integrator Initial condition source : Integrator  InitialConditionSource=external
  Math Function : Math  Operator=pow  SaturateOnIntegerOverflow=on
  Math Function1 : Math  Operator=square  SaturateOnIntegerOverflow=on
  Product1 : Product
  Product2 : Product
  Product3 : Product  Inputs=3
  Product4 : Product
  R_off : Constant  Value=20000
  R_on : Constant  Value=100
  R_on1 : Constant  Value=100
  Switch : Switch  Threshold=1
  Switch1 : Switch
  V-t : Scope
  p : Constant  Value=10
  x-t : Scope
  x0 : Constant  Value=0.7
  𝜇_𝑣 : Constant  Value=10^(-14)
  Out2 : Outport
  wires:
  Constant9/1 -> Switch/1
  Switch/1 -> Switch1/2, Switch1/1
  R_on/1 -> Divide1/1
  Integrator Initial condition source/1 -> Switch/3, Switch/2, x-t/1
  Integrator/1 -> Divide/1, Product4/2
  2p/1 -> Math Function/2
  Divide/1 -> I-t/1, Product3/1
  Switch1/1 -> Product2/2, Add/1, 2x/1
  𝜇_𝑣/1 -> Divide1/2
  Gain2/1 -> Integrator/1
  Math Function/1 -> Add3/2
  Add/1 -> Product1/1
  R_on1/1 -> Product2/1
  Constant/1 -> Add/2
  p/1 -> 2p/1
  D/1 -> Math Function1/1
  Divide1/1 -> Product3/3
  2x/1 -> Add2/2
  Product1/1 -> Add1/2
  R_off/1 -> Product1/2
  Add2/1 -> Math Function/1
  Constant4/1 -> Add3/1, Add2/1
  Product4/1 -> Out2/1, V-t/1
  Product2/1 -> Add1/1
  x0/1 -> Integrator Initial condition source/2
  Constant10/1 -> Switch1/3
  Product3/1 -> Integrator Initial condition source/1
  Add1/1 -> Divide/2
  Add3/1 -> Product3/2
  Math Function1/1 -> Divide1/3
  " V"/1 -> Add4/2
  In1/1 -> Add4/1
  Add4/1 -> Product4/1, Gain2/1

== system memristors_LSTM/Subsystem/Memristor crossbar1/Subsystem15 ==
  note: Memristor
  note: k
  note: for I-V
  note: Rmem
  note: f(x)
  note: for x
  note: for processing
  " V" : Sin  Amplitude=0.1  Frequency=0.5  SampleTime=0
  2p : Gain  Gain=2
  2x : Gain  Gain=2
  Add : Sum  Inputs=-+
  Add1 : Sum
  Add2 : Sum  Inputs=-+
  Add3 : Sum  Inputs=+-
  Constant : Constant
  Constant10 : Constant  Value=0
  Constant4 : Constant
  Constant9 : Constant
  D : Constant  Value=10^(-8)
  Divide : Product  Inputs=*/
  Divide1 : Product  Inputs=**/
  Gain2 : Gain  Gain=0.5
  I-t : Scope
  Integrator : Integrator
  Integrator Initial condition source : Integrator  InitialConditionSource=external
  Math Function : Math  Operator=pow  SaturateOnIntegerOverflow=on
  Math Function1 : Math  Operator=square  SaturateOnIntegerOverflow=on
  Product1 : Product
  Product2 : Product
  Product3 : Product  Inputs=3
  Product4 : Product
  R_off : Constant  Value=20000
  R_on : Constant  Value=100
  R_on1 : Constant  Value=100
  Switch : Switch  Threshold=1
  Switch1 : Switch
  V-t : Scope
  p : Constant  Value=10
  x-t : Scope
  x0 : Constant  Value=0.7
  𝜇_𝑣 : Constant  Value=10^(-14)
  Out1 : Outport
  Out2 : Outport  Port=2
  wires:
  Constant9/1 -> Switch/1
  Switch/1 -> Switch1/2, Switch1/1
  R_on/1 -> Divide1/1
  Integrator Initial condition source/1 -> Switch/3, Switch/2, x-t/1
  Integrator/1 -> Divide/1, Product4/2
  2p/1 -> Math Function/2
  Divide/1 -> I-t/1, Product3/1
  Switch1/1 -> Product2/2, Add/1, 2x/1
  𝜇_𝑣/1 -> Divide1/2
  Gain2/1 -> Integrator/1
  Math Function/1 -> Add3/2
  Add/1 -> Product1/1
  R_on1/1 -> Product2/1
  Constant/1 -> Add/2
  p/1 -> 2p/1
  D/1 -> Math Function1/1
  Divide1/1 -> Product3/3
  2x/1 -> Add2/2
  Product1/1 -> Add1/2
  R_off/1 -> Product1/2
  Add2/1 -> Math Function/1
  Constant4/1 -> Add3/1, Add2/1
  Product4/1 -> Out1/1, Out2/1, V-t/1
  Product2/1 -> Add1/1
  x0/1 -> Integrator Initial condition source/2
  Constant10/1 -> Switch1/3
  Product3/1 -> Integrator Initial condition source/1
  Add1/1 -> Divide/2
  Add3/1 -> Product3/2
  Math Function1/1 -> Divide1/3
  " V"/1 -> Gain2/1, Product4/1

== system memristors_LSTM/Subsystem/Memristor crossbar1/Subsystem16 ==
  note: Memristor
  note: k
  note: for I-V
  note: Rmem
  note: f(x)
  note: for x
  note: for processing
  In1 : Inport
  " V" : Sin  Frequency=0.5  SampleTime=0
  2p : Gain  Gain=2
  2x : Gain  Gain=2
  Add : Sum  Inputs=-+
  Add1 : Sum
  Add2 : Sum  Inputs=-+
  Add3 : Sum  Inputs=+-
  Add4 : Sum
  Constant : Constant
  Constant10 : Constant  Value=0
  Constant4 : Constant
  Constant9 : Constant
  D : Constant  Value=10^(-8)
  Divide : Product  Inputs=*/
  Divide1 : Product  Inputs=**/
  Gain2 : Gain  Gain=0.5
  I-t : Scope
  Integrator : Integrator
  Integrator Initial condition source : Integrator  InitialConditionSource=external
  Math Function : Math  Operator=pow  SaturateOnIntegerOverflow=on
  Math Function1 : Math  Operator=square  SaturateOnIntegerOverflow=on
  Product1 : Product
  Product2 : Product
  Product3 : Product  Inputs=3
  Product4 : Product
  R_off : Constant  Value=20000
  R_on : Constant  Value=100
  R_on1 : Constant  Value=100
  Switch : Switch  Threshold=1
  Switch1 : Switch
  V-t : Scope
  p : Constant  Value=10
  x-t : Scope
  x0 : Constant  Value=0.7
  𝜇_𝑣 : Constant  Value=10^(-14)
  Out1 : Outport
  Out2 : Outport  Port=2
  wires:
  Constant9/1 -> Switch/1
  Switch/1 -> Switch1/2, Switch1/1
  R_on/1 -> Divide1/1
  Integrator Initial condition source/1 -> Switch/3, Switch/2, x-t/1
  2p/1 -> Math Function/2
  Divide/1 -> I-t/1, Product3/1
  Switch1/1 -> Product2/2, Add/1, 2x/1
  𝜇_𝑣/1 -> Divide1/2
  Gain2/1 -> Integrator/1
  Math Function/1 -> Add3/2
  Add/1 -> Product1/1
  R_on1/1 -> Product2/1
  Constant/1 -> Add/2
  p/1 -> 2p/1
  D/1 -> Math Function1/1
  Divide1/1 -> Product3/3
  2x/1 -> Add2/2
  Product1/1 -> Add1/2
  R_off/1 -> Product1/2
  Add2/1 -> Math Function/1
  Constant4/1 -> Add3/1, Add2/1
  Product4/1 -> Out1/1, Out2/1, V-t/1
  Product2/1 -> Add1/1
  x0/1 -> Integrator Initial condition source/2
  Constant10/1 -> Switch1/3
  Product3/1 -> Integrator Initial condition source/1
  Add1/1 -> Divide/2
  Add3/1 -> Product3/2
  Math Function1/1 -> Divide1/3
  " V"/1 -> Add4/2
  In1/1 -> Add4/1
  Add4/1 -> Product4/1, Gain2/1
  Integrator/1 -> Divide/1, Product4/2

== system memristors_LSTM/Subsystem/Memristor crossbar1/Subsystem17 ==
  note: k
  note: for I-V
  note: Rmem
  note: f(x)
  note: for x
  note: for processing
  In1 : Inport
  " V" : Sin  Frequency=0.5  SampleTime=0
  2p : Gain  Gain=2
  2x : Gain  Gain=2
  Add : Sum  Inputs=-+
  Add1 : Sum
  Add2 : Sum  Inputs=-+
  Add3 : Sum  Inputs=+-
  Add4 : Sum
  Constant : Constant
  Constant10 : Constant  Value=0
  Constant4 : Constant
  Constant9 : Constant
  D : Constant  Value=10^(-8)
  Divide : Product  Inputs=*/
  Divide1 : Product  Inputs=**/
  Gain2 : Gain  Gain=0.5
  I-t : Scope
  Integrator : Integrator
  Integrator Initial condition source : Integrator  InitialConditionSource=external
  Math Function : Math  Operator=pow  SaturateOnIntegerOverflow=on
  Math Function1 : Math  Operator=square  SaturateOnIntegerOverflow=on
  Product1 : Product
  Product2 : Product
  Product3 : Product  Inputs=3
  Product4 : Product
  R_off : Constant  Value=20000
  R_on : Constant  Value=100
  R_on1 : Constant  Value=100
  Switch : Switch  Threshold=1
  Switch1 : Switch
  V-t : Scope
  XY Graph : simulink/Sinks/XY Graph  xmin=-1  xmax=1  ymin=-1  ymax=1  st=-1
  p : Constant  Value=10
  x-t : Scope
  x0 : Constant  Value=0.7
  𝜇_𝑣 : Constant  Value=10^(-14)
  Out1 : Outport
  Out2 : Outport  Port=2
  wires:
  Constant9/1 -> Switch/1
  Switch/1 -> Switch1/2, Switch1/1
  R_on/1 -> Divide1/1
  Integrator Initial condition source/1 -> Switch/3, Switch/2, x-t/1
  Integrator/1 -> Divide/1, Product4/2
  2p/1 -> Math Function/2
  Divide/1 -> I-t/1, Product3/1, XY Graph/2
  Switch1/1 -> Product2/2, Add/1, 2x/1
  𝜇_𝑣/1 -> Divide1/2
  Gain2/1 -> Integrator/1
  Math Function/1 -> Add3/2
  Add/1 -> Product1/1
  R_on1/1 -> Product2/1
  Constant/1 -> Add/2
  p/1 -> 2p/1
  D/1 -> Math Function1/1
  Divide1/1 -> Product3/3
  2x/1 -> Add2/2
  Product1/1 -> Add1/2
  R_off/1 -> Product1/2
  Add2/1 -> Math Function/1
  Constant4/1 -> Add3/1, Add2/1
  Product2/1 -> Add1/1
  x0/1 -> Integrator Initial condition source/2
  Constant10/1 -> Switch1/3
  Product3/1 -> Integrator Initial condition source/1
  Add1/1 -> Divide/2
  Add3/1 -> Product3/2
  Math Function1/1 -> Divide1/3
  " V"/1 -> Add4/2
  In1/1 -> Add4/1
  Add4/1 -> Product4/1, Gain2/1
  Product4/1 -> XY Graph/1, Out1/1, Out2/1, V-t/1

== system memristors_LSTM/Subsystem/Memristor crossbar1/Subsystem18 ==
  note: Memristor
  note: k
  note: for I-V
  note: Rmem
  note: f(x)
  note: for x
  note: for processing
  In1 : Inport
  " V" : Sin  Frequency=0.5  SampleTime=0
  2p : Gain  Gain=2
  2x : Gain  Gain=2
  Add : Sum  Inputs=-+
  Add1 : Sum
  Add2 : Sum  Inputs=-+
  Add3 : Sum  Inputs=+-
  Add4 : Sum
  Constant : Constant
  Constant10 : Constant  Value=0
  Constant4 : Constant
  Constant9 : Constant
  D : Constant  Value=10^(-8)
  Divide : Product  Inputs=*/
  Divide1 : Product  Inputs=**/
  Gain2 : Gain  Gain=0.5
  I-t : Scope
  Integrator : Integrator
  Integrator Initial condition source : Integrator  InitialConditionSource=external
  Math Function : Math  Operator=pow  SaturateOnIntegerOverflow=on
  Math Function1 : Math  Operator=square  SaturateOnIntegerOverflow=on
  Product1 : Product
  Product2 : Product
  Product3 : Product  Inputs=3
  Product4 : Product
  R_off : Constant  Value=20000
  R_on : Constant  Value=100
  R_on1 : Constant  Value=100
  Switch : Switch  Threshold=1
  Switch1 : Switch
  V-t : Scope
  p : Constant  Value=10
  x-t : Scope
  x0 : Constant  Value=0.7
  𝜇_𝑣 : Constant  Value=10^(-14)
  Out1 : Outport
  Out2 : Outport  Port=2
  wires:
  Constant9/1 -> Switch/1
  Switch/1 -> Switch1/2, Switch1/1
  R_on/1 -> Divide1/1
  Integrator Initial condition source/1 -> Switch/3, Switch/2, x-t/1
  Integrator/1 -> Divide/1, Product4/2
  2p/1 -> Math Function/2
  Divide/1 -> I-t/1, Product3/1
  Switch1/1 -> Product2/2, Add/1, 2x/1
  𝜇_𝑣/1 -> Divide1/2
  Gain2/1 -> Integrator/1
  Math Function/1 -> Add3/2
  Add/1 -> Product1/1
  R_on1/1 -> Product2/1
  Constant/1 -> Add/2
  p/1 -> 2p/1
  D/1 -> Math Function1/1
  Divide1/1 -> Product3/3
  2x/1 -> Add2/2
  Product1/1 -> Add1/2
  R_off/1 -> Product1/2
  Add2/1 -> Math Function/1
  Constant4/1 -> Add3/1, Add2/1
  Product4/1 -> Out1/1, Out2/1, V-t/1
  Product2/1 -> Add1/1
  x0/1 -> Integrator Initial condition source/2
  Constant10/1 -> Switch1/3
  Product3/1 -> Integrator Initial condition source/1
  Add1/1 -> Divide/2
  Add3/1 -> Product3/2
  Math Function1/1 -> Divide1/3
  " V"/1 -> Add4/2
  In1/1 -> Add4/1
  Add4/1 -> Product4/1, Gain2/1

== system memristors_LSTM/Subsystem/Memristor crossbar1/Subsystem19 ==
  note: Memristor
  note: k
  note: for I-V
  note: Rmem
  note: f(x)
  note: for x
  note: for processing
  In1 : Inport
  " V" : Sin  Frequency=0.5  SampleTime=0
  2p : Gain  Gain=2
  2x : Gain  Gain=2
  Add : Sum  Inputs=-+
  Add1 : Sum
  Add2 : Sum  Inputs=-+
  Add3 : Sum  Inputs=+-
  Add4 : Sum
  Constant : Constant
  Constant10 : Constant  Value=0
  Constant4 : Constant
  Constant9 : Constant
  D : Constant  Value=10^(-8)
  Divide : Product  Inputs=*/
  Divide1 : Product  Inputs=**/
  Gain2 : Gain  Gain=0.5
  I-t : Scope
  Integrator : Integrator
  Integrator Initial condition source : Integrator  InitialConditionSource=external
  Math Function : Math  Operator=pow  SaturateOnIntegerOverflow=on
  Math Function1 : Math  Operator=square  SaturateOnIntegerOverflow=on
  Product1 : Product
  Product2 : Product
  Product3 : Product  Inputs=3
  Product4 : Product
  R_off : Constant  Value=20000
  R_on : Constant  Value=100
  R_on1 : Constant  Value=100
  Switch : Switch  Threshold=1
  Switch1 : Switch
  V-t : Scope
  p : Constant  Value=10
  x-t : Scope
  x0 : Constant  Value=0.7
  𝜇_𝑣 : Constant  Value=10^(-14)
  Out2 : Outport
  wires:
  Constant9/1 -> Switch/1
  Switch/1 -> Switch1/2, Switch1/1
  R_on/1 -> Divide1/1
  Integrator Initial condition source/1 -> Switch/3, Switch/2, x-t/1
  Integrator/1 -> Divide/1, Product4/2
  2p/1 -> Math Function/2
  Divide/1 -> I-t/1, Product3/1
  Switch1/1 -> Product2/2, Add/1, 2x/1
  𝜇_𝑣/1 -> Divide1/2
  Gain2/1 -> Integrator/1
  Math Function/1 -> Add3/2
  Add/1 -> Product1/1
  R_on1/1 -> Product2/1
  Constant/1 -> Add/2
  p/1 -> 2p/1
  D/1 -> Math Function1/1
  Divide1/1 -> Product3/3
  2x/1 -> Add2/2
  Product1/1 -> Add1/2
  R_off/1 -> Product1/2
  Add2/1 -> Math Function/1
  Constant4/1 -> Add3/1, Add2/1
  Product4/1 -> Out2/1, V-t/1
  Product2/1 -> Add1/1
  x0/1 -> Integrator Initial condition source/2
  Constant10/1 -> Switch1/3
  Product3/1 -> Integrator Initial condition source/1
  Add1/1 -> Divide/2
  Add3/1 -> Product3/2
  Math Function1/1 -> Divide1/3
  " V"/1 -> Add4/2
  In1/1 -> Add4/1
  Add4/1 -> Product4/1, Gain2/1

== system memristors_LSTM/Subsystem/Memristor crossbar1/Subsystem2 ==
  note: Memristor
  note: k
  note: for I-V
  note: Rmem
  note: f(x)
  note: for x
  note: for processing
  In1 : Inport
  " V" : Sin  Frequency=0.5  SampleTime=0
  2p : Gain  Gain=2
  2x : Gain  Gain=2
  Add : Sum  Inputs=-+
  Add1 : Sum
  Add2 : Sum  Inputs=-+
  Add3 : Sum  Inputs=+-
  Add4 : Sum
  Constant : Constant
  Constant10 : Constant  Value=0
  Constant4 : Constant
  Constant9 : Constant
  D : Constant  Value=10^(-8)
  Divide : Product  Inputs=*/
  Divide1 : Product  Inputs=**/
  Gain2 : Gain  Gain=0.5
  I-t : Scope
  Integrator : Integrator
  Integrator Initial condition source : Integrator  InitialConditionSource=external
  Math Function : Math  Operator=pow  SaturateOnIntegerOverflow=on
  Math Function1 : Math  Operator=square  SaturateOnIntegerOverflow=on
  Math Function2 : Math  Operator=reciprocal  SaturateOnIntegerOverflow=on
  Product1 : Product
  Product2 : Product
  Product3 : Product  Inputs=3
  Product4 : Product
  R_off : Constant  Value=19360
  R_on : Constant  Value=96
  R_on1 : Constant  Value=87
  Switch : Switch  Threshold=1
  Switch1 : Switch
  V-t : Scope
  p : Constant  Value=10
  x-t : Scope
  x0 : Constant  Value=0.7
  𝜇_𝑣 : Constant  Value=10^(-14)
  Out1 : Outport
  Out2 : Outport  Port=2
  wires:
  Constant9/1 -> Switch/1
  Switch/1 -> Switch1/2, Switch1/1
  R_on/1 -> Divide1/1
  Integrator Initial condition source/1 -> Switch/3, Switch/2, x-t/1
  2p/1 -> Math Function/2
  Divide/1 -> I-t/1, Product3/1
  Switch1/1 -> Product2/2, Add/1, 2x/1
  𝜇_𝑣/1 -> Divide1/2
  Gain2/1 -> Integrator/1
  Math Function/1 -> Add3/2
  Add/1 -> Product1/1
  R_on1/1 -> Product2/1
  Constant/1 -> Add/2
  p/1 -> 2p/1
  D/1 -> Math Function1/1
  Divide1/1 -> Product3/3
  2x/1 -> Add2/2
  Product1/1 -> Add1/2
  R_off/1 -> Product1/2
  Add2/1 -> Math Function/1
  Constant4/1 -> Add3/1, Add2/1
  Product4/1 -> Out2/1, V-t/1
  Product2/1 -> Add1/1
  x0/1 -> Integrator Initial condition source/2
  Constant10/1 -> Switch1/3
  Product3/1 -> Integrator Initial condition source/1
  Add1/1 -> Math Function2/1, Divide/2
  Add3/1 -> Product3/2
  Math Function1/1 -> Divide1/3
  " V"/1 -> Add4/2
  In1/1 -> Add4/1
  Add4/1 -> Product4/1, Gain2/1
  Integrator/1 -> Divide/1, Product4/2
  Math Function2/1 -> Out1/1

== system memristors_LSTM/Subsystem/Memristor crossbar1/Subsystem20 ==
  note: Memristor
  note: k
  note: for I-V
  note: Rmem
  note: f(x)
  note: for x
  note: for processing
  " V" : Sin  Amplitude=0.1  Frequency=0.5  SampleTime=0
  2p : Gain  Gain=2
  2x : Gain  Gain=2
  Add : Sum  Inputs=-+
  Add1 : Sum
  Add2 : Sum  Inputs=-+
  Add3 : Sum  Inputs=+-
  Constant : Constant
  Constant10 : Constant  Value=0
  Constant4 : Constant
  Constant9 : Constant
  D : Constant  Value=10^(-8)
  Divide : Product  Inputs=*/
  Divide1 : Product  Inputs=**/
  Gain2 : Gain  Gain=0.5
  I-t : Scope
  Integrator : Integrator
  Integrator Initial condition source : Integrator  InitialConditionSource=external
  Math Function : Math  Operator=pow  SaturateOnIntegerOverflow=on
  Math Function1 : Math  Operator=square  SaturateOnIntegerOverflow=on
  Product1 : Product
  Product2 : Product
  Product3 : Product  Inputs=3
  Product4 : Product
  R_off : Constant  Value=20000
  R_on : Constant  Value=100
  R_on1 : Constant  Value=100
  Switch : Switch  Threshold=1
  Switch1 : Switch
  V-t : Scope
  p : Constant  Value=10
  x-t : Scope
  x0 : Constant  Value=0.7
  𝜇_𝑣 : Constant  Value=10^(-14)
  Out1 : Outport
  Out2 : Outport  Port=2
  wires:
  Constant9/1 -> Switch/1
  Switch/1 -> Switch1/2, Switch1/1
  R_on/1 -> Divide1/1
  Integrator Initial condition source/1 -> Switch/3, Switch/2, x-t/1
  Integrator/1 -> Divide/1, Product4/2
  2p/1 -> Math Function/2
  Divide/1 -> I-t/1, Product3/1
  Switch1/1 -> Product2/2, Add/1, 2x/1
  𝜇_𝑣/1 -> Divide1/2
  Gain2/1 -> Integrator/1
  Math Function/1 -> Add3/2
  Add/1 -> Product1/1
  R_on1/1 -> Product2/1
  Constant/1 -> Add/2
  p/1 -> 2p/1
  D/1 -> Math Function1/1
  Divide1/1 -> Product3/3
  2x/1 -> Add2/2
  Product1/1 -> Add1/2
  R_off/1 -> Product1/2
  Add2/1 -> Math Function/1
  Constant4/1 -> Add3/1, Add2/1
  Product4/1 -> Out1/1, Out2/1, V-t/1
  Product2/1 -> Add1/1
  x0/1 -> Integrator Initial condition source/2
  Constant10/1 -> Switch1/3
  Product3/1 -> Integrator Initial condition source/1
  Add1/1 -> Divide/2
  Add3/1 -> Product3/2
  Math Function1/1 -> Divide1/3
  " V"/1 -> Gain2/1, Product4/1

== system memristors_LSTM/Subsystem/Memristor crossbar1/Subsystem21 ==
  note: Memristor
  note: k
  note: for I-V
  note: Rmem
  note: f(x)
  note: for x
  note: for processing
  In1 : Inport
  " V" : Sin  Amplitude=0.1  Frequency=0.5  SampleTime=0
  2p : Gain  Gain=2
  2x : Gain  Gain=2
  Add : Sum  Inputs=-+
  Add1 : Sum
  Add2 : Sum  Inputs=-+
  Add3 : Sum  Inputs=+-
  Add4 : Sum
  Constant : Constant
  Constant10 : Constant  Value=0
  Constant4 : Constant
  Constant9 : Constant
  D : Constant  Value=10^(-8)
  Divide : Product  Inputs=*/
  Divide1 : Product  Inputs=**/
  Gain2 : Gain  Gain=0.5
  I-t : Scope
  Integrator : Integrator
  Integrator Initial condition source : Integrator  InitialConditionSource=external
  Math Function : Math  Operator=pow  SaturateOnIntegerOverflow=on
  Math Function1 : Math  Operator=square  SaturateOnIntegerOverflow=on
  Product1 : Product
  Product2 : Product
  Product3 : Product  Inputs=3
  Product4 : Product
  R_off : Constant  Value=20000
  R_on : Constant  Value=100
  R_on1 : Constant  Value=100
  Switch : Switch  Threshold=1
  Switch1 : Switch
  V-t : Scope
  p : Constant  Value=10
  x-t : Scope
  x0 : Constant  Value=0.7
  𝜇_𝑣 : Constant  Value=10^(-14)
  Out1 : Outport
  Out2 : Outport  Port=2
  wires:
  Constant9/1 -> Switch/1
  Switch/1 -> Switch1/2, Switch1/1
  R_on/1 -> Divide1/1
  Integrator Initial condition source/1 -> Switch/3, Switch/2, x-t/1
  2p/1 -> Math Function/2
  Divide/1 -> I-t/1, Product3/1
  Switch1/1 -> Product2/2, Add/1, 2x/1
  𝜇_𝑣/1 -> Divide1/2
  Gain2/1 -> Integrator/1
  Math Function/1 -> Add3/2
  Add/1 -> Product1/1
  R_on1/1 -> Product2/1
  Constant/1 -> Add/2
  p/1 -> 2p/1
  D/1 -> Math Function1/1
  Divide1/1 -> Product3/3
  2x/1 -> Add2/2
  Product1/1 -> Add1/2
  R_off/1 -> Product1/2
  Add2/1 -> Math Function/1
  Constant4/1 -> Add3/1, Add2/1
  Product4/1 -> Out1/1, Out2/1, V-t/1
  Product2/1 -> Add1/1
  x0/1 -> Integrator Initial condition source/2
  Constant10/1 -> Switch1/3
  Product3/1 -> Integrator Initial condition source/1
  Add1/1 -> Divide/2
  Add3/1 -> Product3/2
  Math Function1/1 -> Divide1/3
  " V"/1 -> Add4/2
  In1/1 -> Add4/1
  Add4/1 -> Product4/1, Gain2/1
  Integrator/1 -> Divide/1, Product4/2
